simulink model "V1_S1"  (R2022b)
settings: Solver=VariableStepAuto  StartTime=0.0  StopTime=60  RelTol=1e-3
libraries: mpcadaslib x1, Solver_SF x1
settings Model: Creator=USER  LastModifiedBy=USER
settings DataIOCC: ReturnWorkspaceOutputs=off

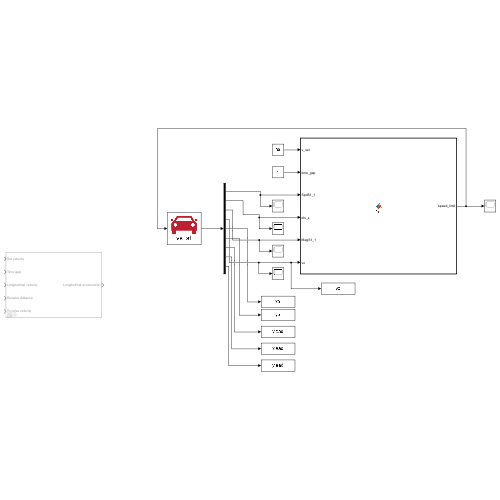
[thumbnail: Simulink's stored preview of the top-level diagram]
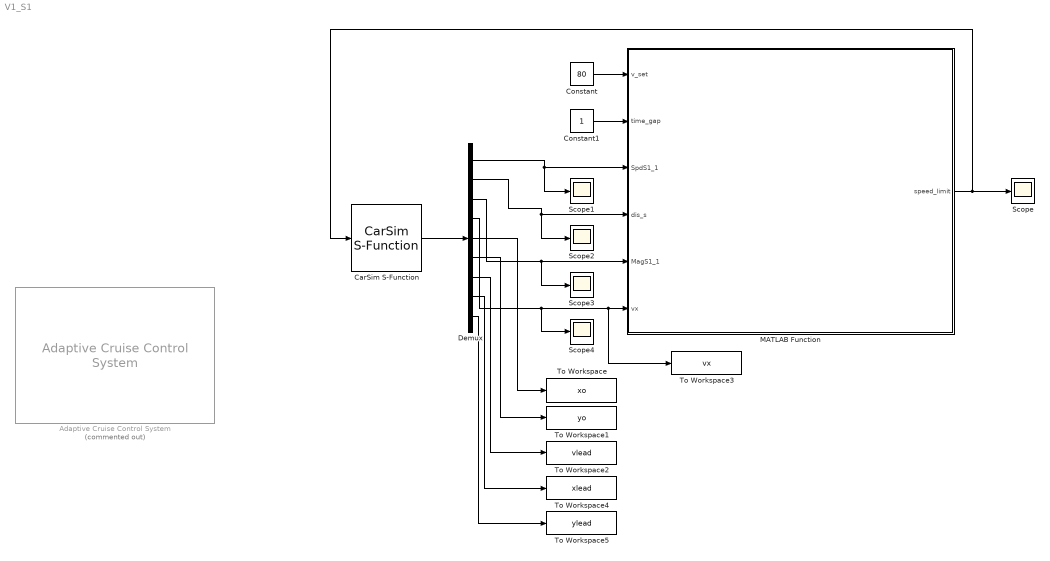
== system V1_S1 ==
  Adaptive Cruise Control System : mpcadaslib/Adaptive Cruise Control System  Commented=on  EgoModel=tf(1,[0.5,1,0])  InitialEgoVelocity=20  DefaultSpacing=10  MaxVelocity=50  MinAcceleration=-3  amin_ext=off  MaxAcceleration=2  amax_ext=off  Ts=0.1  PredictionHorizon=30  ControllerBehavior=0.5  suboptimal=off  maxiter=10  datatypeopt=double  optmode=off  trackmode=off
      settings: LibrarySourceBlock=mpclib/Automated Driving/Adaptive Cruise Control System
  CarSim S-Function : Solver_SF/CarSim S-Function  Priority=1  SIMFILE=simfile.sim  Run_RTs=off  vs_state_ind=Run  StopMode_ind=Vehicle Model
  Constant : Constant  Value=80
  Constant1 : Constant
  Demux : Demux  Outputs=9
  MATLAB Function : MATLAB Function  TreatAsAtomicUnit=on
  Scope{,1..4} (5 alike) : Scope
  To Workspace : ToWorkspace  VariableName=xo  SampleTime=-1
  To Workspace1 : ToWorkspace  VariableName=yo  SampleTime=-1
  To Workspace2 : ToWorkspace  VariableName=vlead  SampleTime=-1
  To Workspace3 : ToWorkspace  VariableName=vx  SampleTime=-1
  To Workspace4 : ToWorkspace  VariableName=xlead  SampleTime=-1
  To Workspace5 : ToWorkspace  VariableName=ylead  SampleTime=-1
  wires:
  CarSim S-Function/1 -> Demux/1
  Constant1/1 -> MATLAB Function/2(time_gap)
  Constant/1 -> MATLAB Function/1(v_set)
  MATLAB Function/1(speed_limit) -> CarSim S-Function/1, Scope/1
  Demux/4 -> Scope4/1, To Workspace3/1, MATLAB Function/6(vx)
  Demux/1 -> Scope1/1, MATLAB Function/3(SpdS1_1)
  Demux/2 -> Scope2/1, MATLAB Function/4(dis_s)
  Demux/3 -> Scope3/1, MATLAB Function/5(MagS1_1)
  Demux/5 -> To Workspace/1
  Demux/6 -> To Workspace1/1
  Demux/7 -> To Workspace2/1
  Demux/8 -> To Workspace4/1
  Demux/9 -> To Workspace5/1

== matlab function V1_S1/MATLAB Function ==
  data: v_set input; time_gap input; speed_limit output; SpdS1_1 input; dis_s input; MagS1_1 input; vx input
function speed_limit  = fcn(v_set,time_gap,SpdS1_1,dis_s,MagS1_1,vx)
vlead=SpdS1_1+vx;
DistanceACC=vlead*time_gap;
if MagS1_1 == 0
    speed_limit=v_set;
else
    a = vx+(SpdS1_1*DistanceACC/dis_s);
    if  a > v_set
        speed_limit=v_set;
    else
        speed_limit = a;
    end
end
